simulink model "untitled2"  (R2015b)
settings: Solver=VariableStepAuto  StartTime=0.0  StopTime=10.0  RelTol=1e-3
values from neighbouring files (symbols this model uses):
  drivefreq = 10e3    (= 10000)    [GE275103.m]    (also in GEWT.m = 5000)
  fluxlinkage = 4    [GE275103.m]    (also in GEWT.m)
  gear = 97    [GEWT.m]
  Jtotal = Jgen+Jtur/(gear^2)    (= 1581.65586141)    [GEWT.m]
  Ld = 10e-4    (= 0.001)    [GE275103.m]    (also in GEWT.m = 0.000248)
  Lq = 10.5e-4    (= 0.00105)    [GE275103.m]    (also in GEWT.m = 0.000292)
  p = 1.225    [GE275103.m]    (also in GEWT.m)
  Prated = 2750000    [GE275103.m]    (also in GEWT.m)
  R = 51.5    [GEWT.m]
  Rs = 1e-10    [GE275103.m]    (also in GEWT.m = 0.0007305)
  Ts = 5E-6    (= 5e-06)    [GE275103.m]    (also in GEWT.m = 1e-05)
  windspeed = 10    [GEWT.m]
libraries: simulink x7, powerlib_meascontrol x7, powerlib x6
settings Model: Creator=Eren  LastModifiedBy=Eren

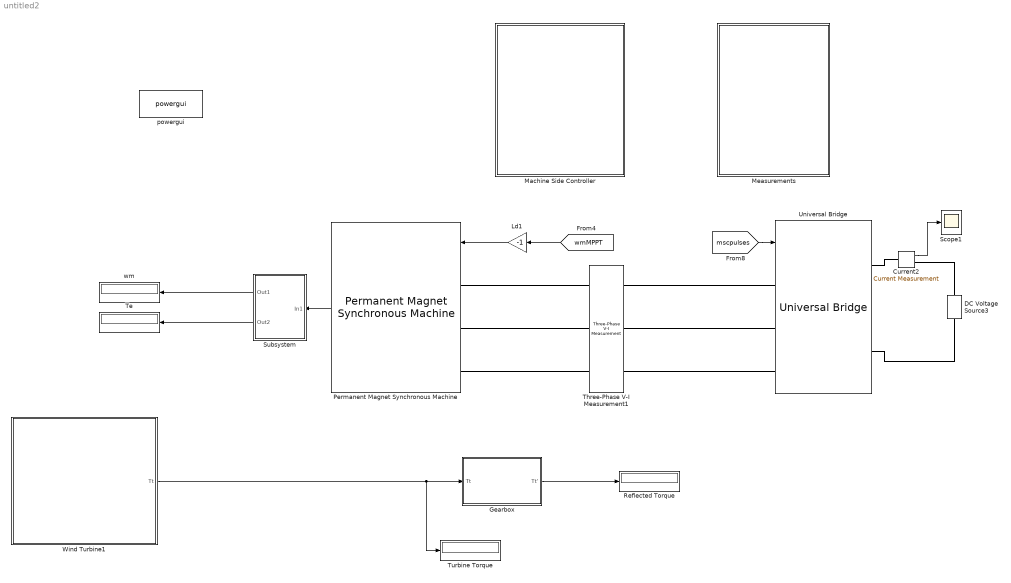
== system untitled2 ==
  Current2 : powerlib/Measurements/Current Measurement  PhasorSimulation=off  OutputType=Complex  PSBequivalent=0
  DC Voltage Source3 : powerlib/Electrical Sources/DC Voltage Source  Amplitude=1200  Measurements=None
  Gearbox : Subsystem
  Ld1 : Gain  Gain=-1
  "Machine Side Controller " : Subsystem
  Measurements : Subsystem
  Permanent Magnet Synchronous Machine : powerlib/Machines/Permanent Magnet Synchronous Machine  NbPhases=3  FluxDistribution=Sinusoidal  RotorType=Salient-pole  MechanicalLoad=Speed w  PresetModel=No  ShowDetailedParameters=on  MeasurementBus=off  Resistance=Rs  Inductance=8.5e-3  dqInductances=[Ld,Lq]  La=0.001764  MachineConstant=Flux linkage established by magnets (V.s)  Flux=1.7933  VoltageCst=650.5373  TorqueCst=5.3799  Flat=120  Mechanical=[Jtotal 1.349e-05 4 0]  PolePairs=2  InitialConditions=[-168.8,0, 0,0]  InitialConditions5ph=[0 0 0 0 0 0]  TsPowergui=0  TsBlock=-1  RefAngle=90 degrees behind phase A axis (modified Park)
  Reflected Torque : Display
  Scope1 : Scope
  Subsystem : Subsystem
  Te : Display
  Three-Phase V-I Measurement1 : powerlib/Measurements/Three-Phase V-I Measurement  VoltageMeasurement=phase-to-phase  SetLabelV=on  LabelV=Vsabc  Vpu=off  VpuLL=on  CurrentMeasurement=yes  SetLabelI=on  LabelI=Isabc  Ipu=on  Pbase=2.75e6  Vbase=690  OutputType=Complex  PhasorSimulation=off  PSBequivalent=0
  Turbine Torque : Display
  Universal Bridge : powerlib/Power Electronics/Universal Bridge  Arms=3  SnubberResistance=1e5  SnubberCapacitance=inf  Device=IGBT / Diodes  Ron=1e-5  Lon=0  ForwardVoltages="[  0  0  ]"  ForwardVoltage=0  GTOparameters=[ 10e-6 , 20e-6 ]  IGBTparameters=[ 1e-6 , 2e-6 ]  Measurements=None  Measurements_2=None  converterType=Rectifier
  Wind Turbine1 : Subsystem
  powergui : powerlib/powergui  Priority=2  SimulationMode=Discrete  SolverType=Tustin  SampleTime=Ts  frequency=60  SPID=off  DisableSnubberDevices=off  DisableRonSwitches=off  DisableVfSwitches=off  SwTol=0  DisplayEquations=off  Interpol=off  ExternalGateDelay=off  methode=off  Ts=0  FunctionMessages=off  echomessages=off  HookPort=off  EnableUseOfTLC=off  x0status=blocks  frequencyindice=0  Pbase=100e6  ErrMax=1e-4  Iterations=50  UnitsV=kV  UnitsW=MW  buscounter=0  RestoreLinks=warning  ResistiveCurrentMeasurement=off  Frange=[0:2:500]  Ylog=off  Xlog=on  ShowGrid=off  save=off  variable=ZData  structure=0  ZoomFFT=on  StartTime=0.0  cycles=1  DisplayStyle=1  fundamental=60  FreqAxis=off  MaxFrequency=1000  frequencyindicesteady=1  RmsSteady=1  display=off
  wm : Display
  wires:
  Current2/1 -> Scope1/1
  Wind Turbine1/1(Tt) -> Turbine Torque/1, Gearbox/1(Tt)
  Gearbox/1(Tt') -> Reflected Torque/1
  Permanent Magnet Synchronous Machine/1 -> Subsystem/1(In1)
  Subsystem/1(Out1) -> wm/1
  Subsystem/2(Out2) -> Te/1
  [mscpulses] -> Universal Bridge/1
  [wmMPPT] -> Ld1/1
  Ld1/1 -> Permanent Magnet Synchronous Machine/1
  connections:
  Three-Phase V-I Measurement1/LConn2 -- Permanent Magnet Synchronous Machine/LConn2
  Three-Phase V-I Measurement1/LConn1 -- Permanent Magnet Synchronous Machine/LConn1
  DC Voltage Source3/RConn1 -- Current2/RConn1
  Three-Phase V-I Measurement1/RConn3 -- Universal Bridge/LConn3
  Permanent Magnet Synchronous Machine/LConn3 -- Three-Phase V-I Measurement1/LConn3
  Universal Bridge/RConn1 -- Current2/LConn1
  Three-Phase V-I Measurement1/RConn1 -- Universal Bridge/LConn1
  Universal Bridge/RConn2 -- DC Voltage Source3/LConn1
  Universal Bridge/LConn2 -- Three-Phase V-I Measurement1/RConn2

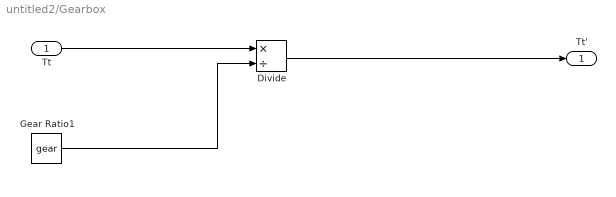
== system untitled2/Gearbox ==
  Tt : Inport
  Divide : Product  Inputs=*/
  Gear Ratio1 : Constant  Value=gear
  Tt' : Outport
  wires:
  Gear Ratio1/1 -> Divide/2
  Tt/1 -> Divide/1
  Divide/1 -> Tt'/1

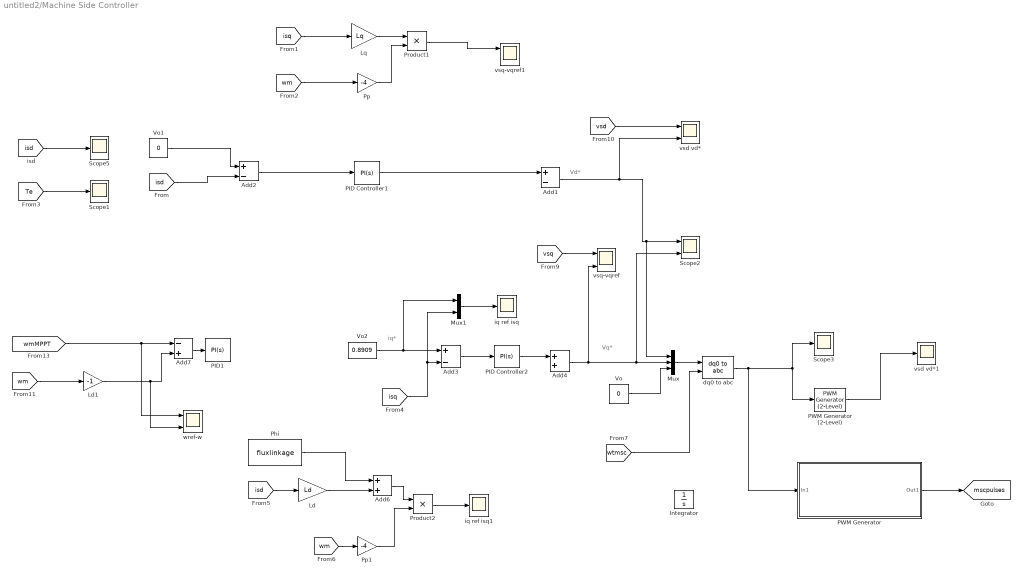
== system untitled2/Machine Side Controller  ==
  note: iq*
  note: Vq*
  note: Vd*
  Add1 : Sum  Inputs=+-
  Add2 : Sum  Inputs=+-
  Add3 : Sum  Inputs=+-
  Add4 : Sum
  Add6 : Sum
  Add7 : Sum  Inputs=-+
  Integrator : Integrator
  Ld : Gain  Gain=Ld
  Ld1 : Gain  Gain=-1
  Lq : Gain  Gain=Lq
  Mux : Mux  Inputs=3
  Mux1 : Mux  Inputs=2
  PID Controller1 : simulink/Continuous/PID Controller  Controller=PI  TimeDomain=Continuous-time  SampleTime=-1  IntegratorMethod=Forward Euler  FilterMethod=Forward Euler  Form=Ideal  UseFilter=on  ControllerParametersSource=internal  P=12.5  I=0.5  D=0  N=100  InitialConditionSource=internal  InitialConditionForIntegrator=0  InitialConditionForFilter=0  ExternalReset=none  LimitOutput=on  UpperSaturationLimit=1  LowerSaturationLimit=-1  LinearizeAsGain=on  AntiWindupMode=none  Kb=1  TrackingMode=off  Kt=1  PParamMin=[]  PParamMax=[]  IParamMin=[]  IParamMax=[]  DParamMin=[]  DParamMax=[]  NParamMin=[]  NParamMax=[]  KbParamMin=[]  KbParamMax=[]  KtParamMin=[]  KtParamMax=[]  POutMin=[]  POutMax=[]  IOutMin=[]  IOutMax=[]  DOutMin=[]  DOutMax=[]  NOutMin=[]  NOutMax=[]  KbOutMin=[]  KbOutMax=[]  KtOutMin=[]  KtOutMax=[]  IntegratorOutMin=[]  IntegratorOutMax=[]  FilterOutMin=[]  FilterOutMax=[]  SumOutMin=[]  SumOutMax=[]  SumI1OutMin=[]  SumI1OutMax=[]  SumI2OutMin=[]  SumI2OutMax=[]  SumI3OutMin=[]  SumI3OutMax=[]  SumDOutMin=[]  SumDOutMax=[]  SaturationOutMin=[]  SaturationOutMax=[]  IntegratorContinuousStateAttributes=''  IntegratorStateMustResolveToSignalObject=off  IntegratorRTWStateStorageClass=Auto  FilterContinuousStateAttributes=''  FilterStateMustResolveToSignalObject=off  FilterRTWStateStorageClass=Auto  DifferentiatorICPrevScaledInput=0  DifferentiatorOutMin=[]  DifferentiatorOutMax=[]
  PID Controller2 : simulink/Continuous/PID Controller  Controller=PI  TimeDomain=Continuous-time  SampleTime=-1  IntegratorMethod=Forward Euler  FilterMethod=Forward Euler  Form=Ideal  UseFilter=on  ControllerParametersSource=internal  P=10  I=0.75  D=0  N=100  InitialConditionSource=internal  InitialConditionForIntegrator=0  InitialConditionForFilter=0  ExternalReset=none  LimitOutput=on  UpperSaturationLimit=1  LowerSaturationLimit=-1  LinearizeAsGain=on  AntiWindupMode=none  Kb=1  TrackingMode=off  Kt=1  PParamMin=[]  PParamMax=[]  IParamMin=[]  IParamMax=[]  DParamMin=[]  DParamMax=[]  NParamMin=[]  NParamMax=[]  KbParamMin=[]  KbParamMax=[]  KtParamMin=[]  KtParamMax=[]  POutMin=[]  POutMax=[]  IOutMin=[]  IOutMax=[]  DOutMin=[]  DOutMax=[]  NOutMin=[]  NOutMax=[]  KbOutMin=[]  KbOutMax=[]  KtOutMin=[]  KtOutMax=[]  IntegratorOutMin=[]  IntegratorOutMax=[]  FilterOutMin=[]  FilterOutMax=[]  SumOutMin=[]  SumOutMax=[]  SumI1OutMin=[]  SumI1OutMax=[]  SumI2OutMin=[]  SumI2OutMax=[]  SumI3OutMin=[]  SumI3OutMax=[]  SumDOutMin=[]  SumDOutMax=[]  SaturationOutMin=[]  SaturationOutMax=[]  IntegratorContinuousStateAttributes=''  IntegratorStateMustResolveToSignalObject=off  IntegratorRTWStateStorageClass=Auto  FilterContinuousStateAttributes=''  FilterStateMustResolveToSignalObject=off  FilterRTWStateStorageClass=Auto  DifferentiatorICPrevScaledInput=0  DifferentiatorOutMin=[]  DifferentiatorOutMax=[]
  PID1 : simulink/Continuous/PID Controller  Controller=PI  TimeDomain=Continuous-time  SampleTime=-1  IntegratorMethod=Forward Euler  FilterMethod=Forward Euler  Form=Ideal  UseFilter=on  ControllerParametersSource=internal  P=0.1  I=1  D=0  N=100  InitialConditionSource=internal  InitialConditionForIntegrator=0  InitialConditionForFilter=0  ExternalReset=none  LimitOutput=on  UpperSaturationLimit=2  LowerSaturationLimit=-2  LinearizeAsGain=on  AntiWindupMode=none  Kb=1  TrackingMode=off  Kt=1  PParamMin=[]  PParamMax=[]  IParamMin=[]  IParamMax=[]  DParamMin=[]  DParamMax=[]  NParamMin=[]  NParamMax=[]  KbParamMin=[]  KbParamMax=[]  KtParamMin=[]  KtParamMax=[]  POutMin=[]  POutMax=[]  IOutMin=[]  IOutMax=[]  DOutMin=[]  DOutMax=[]  NOutMin=[]  NOutMax=[]  KbOutMin=[]  KbOutMax=[]  KtOutMin=[]  KtOutMax=[]  IntegratorOutMin=[]  IntegratorOutMax=[]  FilterOutMin=[]  FilterOutMax=[]  SumOutMin=[]  SumOutMax=[]  SumI1OutMin=[]  SumI1OutMax=[]  SumI2OutMin=[]  SumI2OutMax=[]  SumI3OutMin=[]  SumI3OutMax=[]  SumDOutMin=[]  SumDOutMax=[]  SaturationOutMin=[]  SaturationOutMax=[]  IntegratorContinuousStateAttributes=''  IntegratorStateMustResolveToSignalObject=off  IntegratorRTWStateStorageClass=Auto  FilterContinuousStateAttributes=''  FilterStateMustResolveToSignalObject=off  FilterRTWStateStorageClass=Auto  DifferentiatorICPrevScaledInput=0  DifferentiatorOutMin=[]  DifferentiatorOutMax=[]
  "PWM Generator " : Subsystem
  PWM Generator (2-Level) : powerlib_meascontrol/Pulse & Signal Generators/PWM Generator (2-Level)  ModulatorType=Three-phase bridge (6 pulses)  ModulatorMode=Unsynchronized  Fc=drivefreq  Pc=90  nF=drivefreq/50  MinMax="[ -1  1 ]"  SamplingTechnique=Natural  ModulatingSignals=off  m=0.8  Freq=60  Phase=0  Ts=Ts  ShowCarrierOutport=off
  Phi : Constant  Value=fluxlinkage
  Pp : Gain  Gain=-4
  Pp1 : Gain  Gain=-4
  Product1 : Product
  Product2 : Product
  Scope1 : Scope
  Scope2 : Scope  NumInputPorts=2
  Scope3 : Scope
  Scope5 : Scope
  Vo : Constant  Value=0
  Vo1 : Constant  Value=0
  Vo2 : Constant  Value=0.8909
  dq0 to abc : powerlib_meascontrol/Transformations/dq0 to abc  Alignment=90 degrees behind phase A axis
  iq ref isq : Scope
  iq ref isq1 : Scope
  vsd vd* : Scope  NumInputPorts=2
  vsd vd*1 : Scope
  vsq-vqref : Scope  NumInputPorts=2
  vsq-vqref1 : Scope  NumInputPorts=2
  wref-w : Scope  NumInputPorts=2
  tag scope: mscpulses=global
  wires:
  [wm] -> Ld1/1
  Mux/1 -> dq0 to abc/1
  Vo1/1 -> Add2/1
  Vo/1 -> Mux/3
  [isq] -> Mux1/2, Add3/2
  [wm] -> Pp1/1
  Add3/1 -> PID Controller2/1
  Add2/1 -> PID Controller1/1
  Pp1/1 -> Product2/2
  Ld/1 -> Add6/2
  [isd] -> Add2/2
  Lq/1 -> Product1/1
  Phi/1 -> Add6/1
  PID Controller1/1 -> Add1/1
  Add6/1 -> Product2/1
  Pp/1 -> Product1/2
  [isd] -> Ld/1
  [wm] -> Pp/1
  Ld1/1 -> wref-w/2, Add7/2
  PID Controller2/1 -> Add4/1
  [isq] -> Lq/1
  [vsq] -> vsq-vqref/1
  [vsd] -> vsd vd*/1
  Mux1/1 -> iq ref isq/1
  Product1/1 -> vsq-vqref1/1
  [isd] -> Scope5/1
  [Te] -> Scope1/1
  PWM Generator (2-Level)/1 -> vsd vd*1/1
  [wmMPPT] -> wref-w/1, Add7/1
  Add1/1 -> Mux/1, Scope2/1, vsd vd*/2
  Add4/1 -> Mux/2, Scope2/2, vsq-vqref/2
  Vo2/1 -> Mux1/1, Add3/1
  Product2/1 -> iq ref isq1/1
  dq0 to abc/1 -> "PWM Generator "/1(In1), PWM Generator (2-Level)/1, Scope3/1
  Add7/1 -> PID1/1
  [wtmsc] -> dq0 to abc/2
  "PWM Generator "/1(Out1) -> [mscpulses]

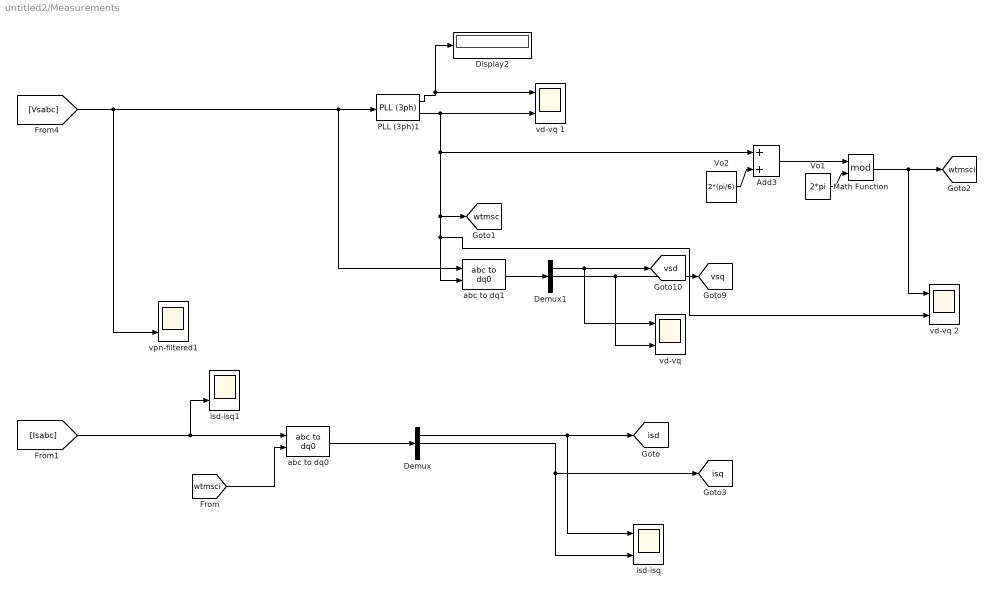
== system untitled2/Measurements ==
  Add3 : Sum
  Demux : Demux  Outputs=3
  Demux1 : Demux  Outputs=3
  Display2 : Display
  Math Function : Math  Operator=mod  SaturateOnIntegerOverflow=on
  PLL (3ph)1 : powerlib_meascontrol/PLL/PLL (3ph)  Fmin=55/3  Par_Init=[0, 50]  ParK=[180, 3200, 1]  TcD=1e-4  MaxRateChangeFreq=100  FilterCutOffFreq=25  Ts=0  AGC=on
  Vo1 : Constant  Value=2*pi
  Vo2 : Constant  Value=2*(pi/6)
  abc to dq0 : powerlib_meascontrol/Transformations/abc to dq0  Alignment=90 degrees behind phase A axis
  abc to dq1 : powerlib_meascontrol/Transformations/abc to dq0  Alignment=90 degrees behind phase A axis
  isd-isq : Scope  NumInputPorts=2
  isd-isq1 : Scope  NumInputPorts=2
  "vd-vq " : Scope  NumInputPorts=2
  vd-vq 1 : Scope  NumInputPorts=2
  vd-vq 2 : Scope  NumInputPorts=2
  vpn-filtered1 : Scope  NumInputPorts=2
  tag scope: isd=global, isq=global, vsd=global, vsq=global, wtmsc=global, wtmsci=global
  wires:
  [Vsabc] -> vpn-filtered1/2, abc to dq1/1, PLL (3ph)1/1
  PLL (3ph)1/1 -> Display2/1, vd-vq 1/1
  [Isabc] -> isd-isq1/2, abc to dq0/1
  abc to dq0/1 -> Demux/1
  abc to dq1/1 -> Demux1/1
  Demux1/1 -> "vd-vq "/1, [vsd]
  Demux1/2 -> "vd-vq "/2, [vsq]
  Demux/1 -> isd-isq/1, [isd]
  Demux/2 -> [isq], isd-isq/2
  Math Function/1 -> vd-vq 2/1, [wtmsci]
  Add3/1 -> Math Function/1
  Vo2/1 -> Add3/2
  Vo1/1 -> Math Function/2
  [wtmsci] -> abc to dq0/2
  PLL (3ph)1/2 -> Add3/1, [wtmsc], vd-vq 2/2, abc to dq1/2, vd-vq 1/2

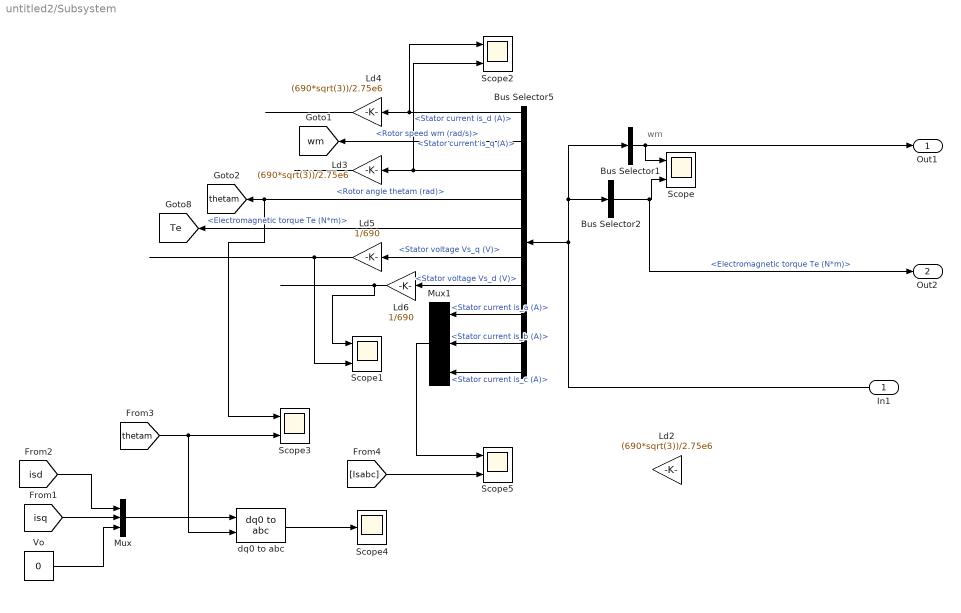
== system untitled2/Subsystem ==
  note: wm
  In1 : Inport
  Bus Selector1 : BusSelector  OutputSignals=Rotor speed wm (rad/s)  OutputAsBus=on
  Bus Selector2 : BusSelector  OutputSignals=Electromagnetic torque Te (N*m)
  Bus Selector5 : BusSelector  OutputSignals=Stator current is_d (A),Rotor speed wm (rad/s),Stator current is_q (A),Rotor angle thetam (rad),Electromagnetic torque Te (N*m),Stator voltage Vs_q (V),Stator voltage Vs_d (V),Stator current is_a (A),Stator current is_b (A),Stator current is_c (A)
  Ld2 : Gain  Gain=(690*sqrt(3))/2.75e6
  Ld3 : Gain  Gain=(690*sqrt(3))/2.75e6
  Ld4 : Gain  Gain=(690*sqrt(3))/2.75e6
  Ld5 : Gain  Gain=1/690
  Ld6 : Gain  Gain=1/690
  Mux : Mux  Inputs=3
  Mux1 : Mux  Inputs=3
  Scope{,1..3,5} (5 alike) : Scope  NumInputPorts=2
  Scope4 : Scope
  Vo : Constant  Value=0
  dq0 to abc : powerlib_meascontrol/Transformations/dq0 to abc  Alignment=Aligned with phase A axis
  Out1 : Outport
  Out2 : Outport  Port=2
  tag scope: Te=global, thetam=global, wm=global
  wires:
  Bus Selector1/1 -> Out1/1, Scope/1
  In1/1 -> Bus Selector1/1, Bus Selector2/1, Bus Selector5/1
  Bus Selector5/1 -> Scope2/1, Ld4/1  "<Stator current is_d (A)>"
  Bus Selector2/1 -> Out2/1, Scope/2  "<Electromagnetic torque Te (N*m)>"
  Bus Selector5/3 -> Scope2/2, Ld3/1  "<Stator current is_q (A)>"
  Bus Selector5/4 -> Scope3/1, [thetam]  "<Rotor angle thetam (rad)>"
  Bus Selector5/5 -> [Te]  "<Electromagnetic torque Te (N*m)>"
  Bus Selector5/6 -> Ld5/1  "<Stator voltage Vs_q (V)>"
  Bus Selector5/7 -> Ld6/1  "<Stator voltage Vs_d (V)>"
  Bus Selector5/2 -> [wm]  "<Rotor speed wm (rad/s)>"
  [thetam] -> Scope3/2, dq0 to abc/2
  Mux/1 -> dq0 to abc/1
  Vo/1 -> Mux/3
  [isd] -> Mux/1
  [isq] -> Mux/2
  dq0 to abc/1 -> Scope4/1
  Bus Selector5/9 -> Mux1/2  "<Stator current is_b (A)>"
  Bus Selector5/10 -> Mux1/3  "<Stator current is_c (A)>"
  Bus Selector5/8 -> Mux1/1  "<Stator current is_a (A)>"
  Mux1/1 -> Scope5/1
  [Isabc] -> Scope5/2
  Ld3/1 -> ?
  Ld4/1 -> ?
  Ld5/1 -> Scope1/2
  Ld6/1 -> Scope1/1

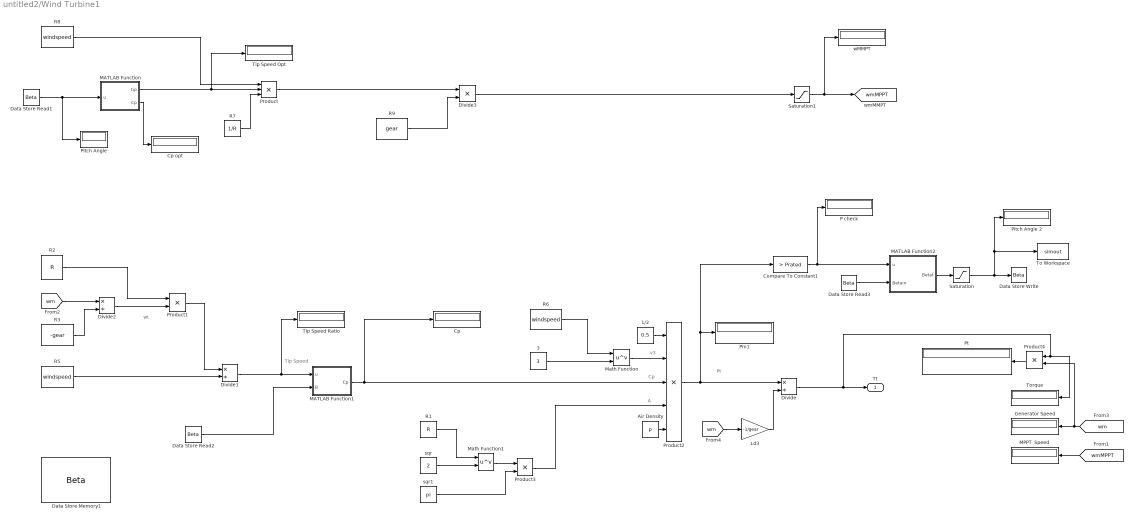
== system untitled2/Wind Turbine1 ==
  note: Pt
  note: v3
  note: Cp
  note: A
  note: wt
  note: Tip Speed
  1/2 : Constant  Value=0.5
  3 : Constant  Value=3
  Air Density : Constant  Value=p
  Compare To Constant1 : simulink/Logic and Bit Operations/Compare To Constant  relop=>  const=Prated  OutDataTypeStr=boolean
  Cp : Display
  Cp opt : Display
  Data Store Memory1 : DataStoreMemory  DataStoreName=Beta  ReadBeforeWriteMsg=warning  WriteAfterWriteMsg=warning  WriteAfterReadMsg=warning  OutMin=[0]  OutMax=[90]
  Data Store Read1 : DataStoreRead  DataStoreName=Beta  SampleTime=Ts
  Data Store Read2 : DataStoreRead  DataStoreName=Beta  SampleTime=Ts
  Data Store Read3 : DataStoreRead  DataStoreName=Beta  SampleTime=Ts
  Data Store Write : DataStoreWrite  DataStoreName=Beta
  Divide : Product  Inputs=*/
  Divide1 : Product  Inputs=*/
  Divide2 : Product  Inputs=*/
  Divide3 : Product  Inputs=**
  Generator Speed : Display
  Ld3 : Gain  Gain=-1/gear
  MATLAB Function : MATLAB Function  TreatAsAtomicUnit=on
  MATLAB Function1 : MATLAB Function  TreatAsAtomicUnit=on
  MATLAB Function2 : MATLAB Function  TreatAsAtomicUnit=on
  MPPT  Speed : Display
  Math Function : Math  Operator=pow  SaturateOnIntegerOverflow=on
  Math Function1 : Math  Operator=pow  SaturateOnIntegerOverflow=on
  P check : Display
  "Pitch Angle " : Display
  Pitch Angle 2 : Display
  Pm1 : Display
  Product : Product  Inputs=3
  Product1 : Product
  Product2 : Product  Inputs=5
  Product3 : Product
  Product4 : Product
  Pt : Display
  R1 : Constant  Value=R
  R2 : Constant  Value=R
  R3 : Constant  Value=-gear
  R5 : Constant  Value=windspeed
  R6 : Constant  Value=windspeed
  R7 : Constant  Value=1/R
  R8 : Constant  Value=windspeed
  R9 : Constant  Value=gear
  Saturation : Saturate  UpperLimit=90  LowerLimit=0
  Saturation1 : Saturate  UpperLimit=181.68  LowerLimit=0
  "Tip Speed Opt " : Display
  "Tip Speed Ratio " : Display
  To Workspace : ToWorkspace  VariableName=simout  SaveFormat=Timeseries  SampleTime=-1
  Torque : Display
  sqr : Constant  Value=2
  sqr1 : Constant  Value=pi
  "wMMPT " : Display
  Tt : Outport
  tag scope: wmMPPT=global
  wires:
  Air Density/1 -> Product2/5
  1/2/1 -> Product2/1
  Product3/1 -> Product2/4
  Math Function1/1 -> Product3/1
  sqr1/1 -> Product3/2
  [wm] -> Ld3/1
  Math Function/1 -> Product2/2
  sqr/1 -> Math Function1/2
  R1/1 -> Math Function1/1
  Product2/1 -> Divide/1, Compare To Constant1/1, Pm1/1
  3/1 -> Math Function/2
  R2/1 -> Product1/1
  [wm] -> Divide2/1
  Product1/1 -> Divide1/1
  R5/1 -> Divide1/2
  Divide1/1 -> MATLAB Function1/1(u), "Tip Speed Ratio "/1
  Divide2/1 -> Product1/2
  Ld3/1 -> Divide/2
  MATLAB Function1/1(Cp) -> Product2/3, Cp/1
  R3/1 -> Divide2/2
  R6/1 -> Math Function/1
  MATLAB Function/1(tip) -> "Tip Speed Opt "/1, Product/2
  R7/1 -> Product/3
  R8/1 -> Product/1
  Product/1 -> Divide3/1
  R9/1 -> Divide3/2
  MATLAB Function/2(Cp) -> Cp opt/1
  Divide3/1 -> Saturation1/1
  Data Store Read3/1 -> MATLAB Function2/2(Betain)
  Data Store Read2/1 -> MATLAB Function1/2(B)
  Data Store Read1/1 -> "Pitch Angle "/1, MATLAB Function/1(u)
  MATLAB Function2/1(Betaf) -> Saturation/1
  Compare To Constant1/1 -> MATLAB Function2/1(u), P check/1
  Saturation/1 -> To Workspace/1, Pitch Angle 2/1, Data Store Write/1
  Saturation1/1 -> "wMMPT "/1, [wmMPPT]
  [wm] -> Generator Speed/1, Product4/2
  Product4/1 -> Pt/1
  Divide/1 -> Product4/1, Torque/1, Tt/1
  [wmMPPT] -> MPPT  Speed/1

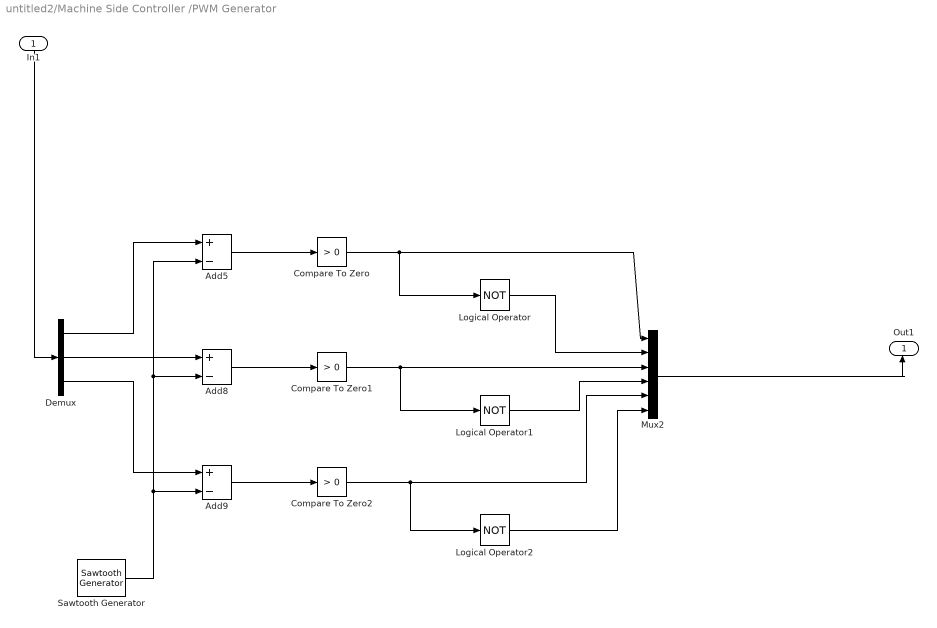
== system untitled2/Machine Side Controller /PWM Generator  ==
  In1 : Inport
  Add5 : Sum  Inputs=+-
  Add8 : Sum  Inputs=+-
  Add9 : Sum  Inputs=+-
  Compare To Zero : simulink/Logic and Bit Operations/Compare To Zero  relop=>  OutDataTypeStr=boolean
  Compare To Zero1 : simulink/Logic and Bit Operations/Compare To Zero  relop=>  OutDataTypeStr=boolean
  Compare To Zero2 : simulink/Logic and Bit Operations/Compare To Zero  relop=>  OutDataTypeStr=boolean
  Demux : Demux  Outputs=3
  Logical Operator : Logic  Operator=NOT  AllPortsSameDT=off  OutDataTypeStr=boolean
  Logical Operator1 : Logic  Operator=NOT  AllPortsSameDT=off  OutDataTypeStr=boolean
  Logical Operator2 : Logic  Operator=NOT  AllPortsSameDT=off  OutDataTypeStr=boolean
  Mux2 : Mux  Inputs=6
  Sawtooth Generator : powerlib_meascontrol/Pulse & Signal Generators/Sawtooth Generator  Freq=drivefreq  Phase=0  Ts=0
  Out1 : Outport
  wires:
  Mux2/1 -> Out1/1
  Add8/1 -> Compare To Zero1/1
  Demux/1 -> Add5/1
  Compare To Zero/1 -> Logical Operator/1, Mux2/1
  Add9/1 -> Compare To Zero2/1
  Demux/2 -> Add8/1
  Demux/3 -> Add9/1
  Logical Operator2/1 -> Mux2/6
  Add5/1 -> Compare To Zero/1
  In1/1 -> Demux/1
  Sawtooth Generator/1 -> Add8/2, Add5/2, Add9/2
  Compare To Zero1/1 -> Logical Operator1/1, Mux2/3
  Logical Operator/1 -> Mux2/2
  Compare To Zero2/1 -> Logical Operator2/1, Mux2/5
  Logical Operator1/1 -> Mux2/4

== matlab function untitled2/Wind Turbine1/MATLAB Function ==
  data: u input; tip output; Cp output
function [tip,Cp]= fcn(u)

c1 = 0.5176;
c2 = 116;
c3 = 0.4;
c4 = 5;
c5 = 21;
c6 = 0.0068;
B=0;
for i = 0.1:0.1:15
    
li = 1/((1/(i+0.08*u))-(0.035/(u^3+1)));
A = c1*((c2/li-c3*u-c4)*exp(-c5/li))+c6*i ;%#codegen

    if A < B
    lopt = i;
    break
    else 
    B = A;
    end
end
tip = i;
Cp = c1*((c2/li-c3*u-c4)*exp(-c5/li))+c6*i;
end

== matlab function untitled2/Wind Turbine1/MATLAB Function1 ==
  data: u input; B input; Cp output
function Cp = fcn(u,B)

c1 = 0.5176;
c2 = 116;
c3 = 0.4; 
c4 = 5;
c5 = 21;
c6 = 0.0068;

i =u;

li = 1/((1/(i+0.08*B))-(0.035/(B^3+1)));

Cp = c1*((c2/li-c3*B-c4)*exp(-c5/li))+c6*i;

end

== matlab function untitled2/Wind Turbine1/MATLAB Function2 ==
  data: u input; Betaf output; Betain input
function Betaf  = fcn(u,Betain)

    if u ==1
    Betaf = Betain+0.01;
    else  

    Betaf = Betain-0.01;
    end
 
    
    
end
